simulink model "example_House_SFH15"  (R2013b)
settings: Solver=ode45  StartTime=-30*24*3600  StopTime=365*24*3600  RelTol=1e-3
libraries: carnot x5, simulink x3
settings Model: SimulationMode=accelerator  Creator=U_13.adm_zivi  LastModifiedBy=drhf
settings DataIOCC: SignalLoggingSaveFormat=ModelDataLogs
settings DebuggingCC: FcnCallInpInsideContextMsg=EnableAllAsWarning
settings GRTTargetCC: CombineOutputUpdateFcns=off  GRTInterface=on

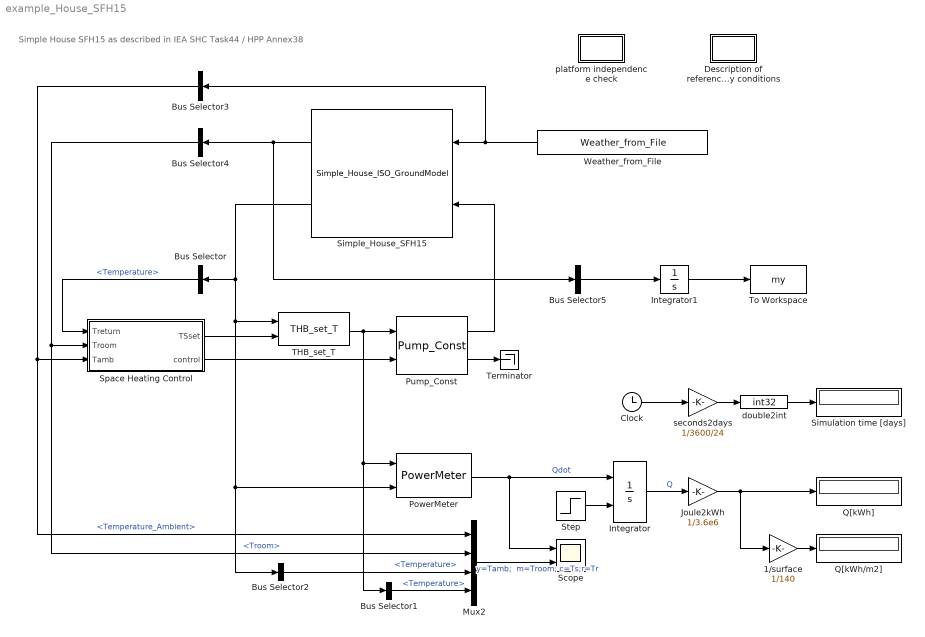
== system example_House_SFH15 ==
  note: Simple House SFH15 as described in IEA SHC Task44 / HPP Annex38
  1/surface : Gain  Gain=1/140
  Bus Selector : BusSelector  OutputSignals=Temperature
  Bus Selector1 : BusSelector  OutputSignals=Temperature
  Bus Selector2 : BusSelector  OutputSignals=Temperature
  Bus Selector3 : BusSelector  OutputSignals=Temperature_Ambient
  Bus Selector4 : BusSelector  OutputSignals=Troom
  Bus Selector5 : BusSelector  OutputSignals=Qdot  OutputAsBus=on
  Clock : Clock
  "Description of reference buidling and boundary conditions " : Subsystem
      settings: OpenFcn=|
      | filepath = fullfile(path_carnot('libsl'),'Load','Houses', 'Simple_House_ISO_GroundModel','specification');
      | 
      | open(fullfile(filepath, 'T44A38_Rep_C1_B_ReferenceBuildingDescription_Final_Revised_130906.pdf'));
      | open(fullfile(filepath, 'T44A38_Rep_C1_A_BoundaryConditions_Final_Revised_131108.pdf'));
      mask Display: disp('.pdf')
  Integrator : Integrator  ExternalReset=rising
  Integrator1 : Integrator
  Joule2kWh : Gain  Gain=1/3.6e6
  Mux2 : Mux
  PowerMeter : carnot/Control/PowerMeter
  Pump_Const : carnot/Hydraulics/Pump_Const  mdotmax=308/3600  dia=0.02  power=81  p0=3e5  fluid_id=Water  mix=0  UA=3  mcp=4000  tamb=20
  Q[kWh/m2] : Display
  Q[kWh] : Display
  Scope : Scope  NumInputPorts=2
      settings: TickLabels=on  YMin=-7.5~0  YMax=35~0.0019  Decimation=1000  SampleInput=on  SampleTime=3600*3
  Simple_House_SFH15 : carnot/Load/Houses/Simple_House_ISO_GroundModel  Ahabit=140  Hroom=2.6  Floorsize=[7 10]  UAwall=0.162*(54.6+26.4)+0.182*((45.7+56.0)*2 -(12+4+3+4))  UAneighbour=0  Uground=0.1  mc=0.5e6*140 % 0.5 MJ/m2/K  shade=0.75  tini=20  Awin=[12 4 3 4]  AziWin=[0 90 -180 -90]  Uwin="[1    1   1    1]*1.0"  Gwin="[1    1   1    1]*0.585*(1-0.15)"  vent=0.4  rec=0.6  heatload=1792  delta_t_nom=15  n_rad=1.1  mass_times_cap=40e6  dpcoeff=[10 100]
  Simulation time [days] : Display
  Space Heating Control : Subsystem  mask{Tset=20, Q_LOC=1792, Td_in=35, Td_out=30, Tambd=-10, n_rad=1.1}
      mask prompts: Tset "desired room Temperature [°C]"; Q_LOC "design heat load [W]"; Td_in "design inlet temperature of the heating system [°C]"; Td_out "design outlet temperature of the heating system [°C]"; Tambd "design outdoor temperature"; n_rad "radiatior exponent"
      mask init:
      | dTd = 0.5*(Td_in + Td_out) - Tset;
  Step : Step  Time=0  SampleTime=0
  THB_set_T : carnot/Source/Simple/THB_set_T
  Terminator : Terminator
  To Workspace : ToWorkspace  VariableName=my  SampleTime=3600
  Weather_from_File : carnot/Weather/Weather_from_File  file=DE_TRY2010_12_averageYear  ext=.mat
  double2int : DataTypeConversion  OutDataTypeStr=int32
  "platform independence check " : Subsystem
      settings: OpenFcn=open(fullfile(path_carnot('help'), 'pdf', 'Peter_Wintler_Dott_IEA_Task_44_Building_2014.pdf'));
      mask Display: disp('.pdf')
  seconds2days : Gain  Gain=1/3600/24
  wires:
  Space Heating Control/1(TSset) -> THB_set_T/2
  Space Heating Control/2(control) -> Pump_Const/2
  Weather_from_File/1 -> Bus Selector3/1, Simple_House_SFH15/1
  Pump_Const/1 -> Simple_House_SFH15/2
  Simple_House_SFH15/2 -> Bus Selector/1, Bus Selector2/1, PowerMeter/2, THB_set_T/1
  Bus Selector/1 -> Space Heating Control/1(Treturn)  "<Temperature>"
  Simple_House_SFH15/1 -> Bus Selector4/1, Bus Selector5/1
  Pump_Const/2 -> Terminator/1
  Bus Selector3/1 -> Space Heating Control/3(Tamb), Mux2/1  "<Temperature_Ambient>"
  Clock/1 -> seconds2days/1
  seconds2days/1 -> double2int/1
  double2int/1 -> Simulation time [days]/1
  Bus Selector2/1 -> Mux2/3  "<Temperature>"
  Bus Selector1/1 -> Mux2/4  "<Temperature>"
  PowerMeter/1 -> Integrator/1, Scope/1  "Qdot"
  1/surface/1 -> Q[kWh/m2]/1
  Integrator/1 -> Joule2kWh/1  "Q"
  THB_set_T/1 -> Bus Selector1/1, PowerMeter/1, Pump_Const/1
  Step/1 -> Integrator/2
  Mux2/1 -> Scope/2  "y=Tamb;  m=Troom; c=Ts;r=Tr"
  Joule2kWh/1 -> 1/surface/1, Q[kWh]/1
  Integrator1/1 -> To Workspace/1
  Bus Selector4/1 -> Mux2/2, Space Heating Control/2(Troom)  "<Troom>"
  Bus Selector5/1 -> Integrator1/1

== system example_House_SFH15/Description of reference buidling and boundary conditions  ==

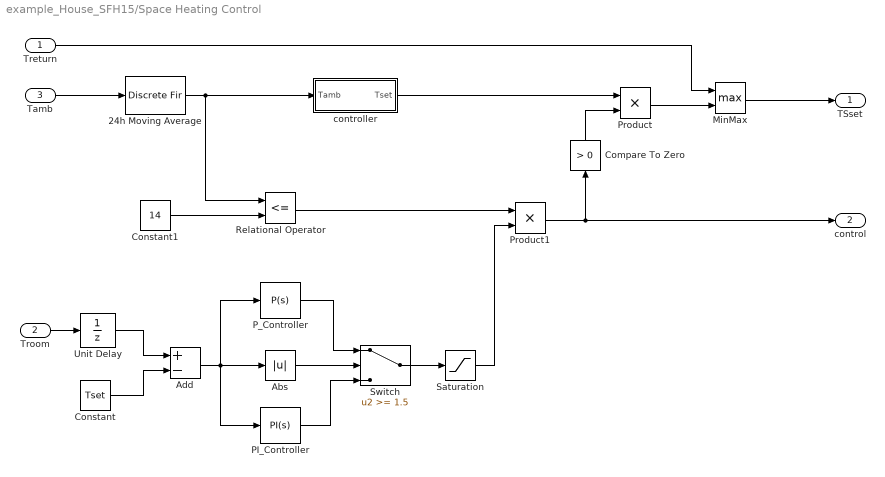
== system example_House_SFH15/Space Heating Control ==
  Treturn : Inport
  Troom : Inport  Port=2
  Tamb : Inport  Port=3
  24h Moving Average : DiscreteFir  Coefficients=ones(1,24)*(1/24)  SampleTime=3600  AccumDataTypeStr=Inherit: Same as product output  RndMeth=Nearest
  Abs : Abs
  Add : Sum  Inputs=+-
  Compare To Zero : simulink/Logic and Bit Operations/Compare To Zero  relop=>  OutDataTypeStr=boolean
  Constant : Constant  Value=Tset
  Constant1 : Constant  Value=14
  MinMax : MinMax  Function=max  Inputs=2
  PI_Controller : simulink/Continuous/PID Controller  Controller=PI  TimeDomain=Continuous-time  SampleTime=1  IntegratorMethod=Forward Euler  FilterMethod=Forward Euler  Form=Parallel  P=-0.8  I=-0.05/3600  D=0  N=100  InitialConditionSource=internal  InitialConditionForIntegrator=0  InitialConditionForFilter=0  ExternalReset=none  ZeroCross=off  LimitOutput=on  UpperSaturationLimit=1  LowerSaturationLimit=0  LinearizeAsGain=off  AntiWindupMode=back-calculation  Kb=1  TrackingMode=off  Kt=1  PParamMin=[]  PParamMax=[]  IParamMin=[]  IParamMax=[]  DParamMin=[]  DParamMax=[]  NParamMin=[]  NParamMax=[]  KbParamMin=[]  KbParamMax=[]  KtParamMin=[]  KtParamMax=[]  POutMin=[]  POutMax=[]  IOutMin=[]  IOutMax=[]  DOutMin=[]  DOutMax=[]  NOutMin=[]  NOutMax=[]  KbOutMin=[]  KbOutMax=[]  KtOutMin=[]  KtOutMax=[]  IntegratorOutMin=[]  IntegratorOutMax=[]  FilterOutMin=[]  FilterOutMax=[]  SumOutMin=[]  SumOutMax=[]  SumI1OutMin=[]  SumI1OutMax=[]  SumI2OutMin=[]  SumI2OutMax=[]  SumI3OutMin=[]  SumI3OutMax=[]  SumDOutMin=[]  SumDOutMax=[]  SaturationOutMin=[]  SaturationOutMax=[]  IntegratorContinuousStateAttributes=''  IntegratorStateMustResolveToSignalObject=off  IntegratorRTWStateStorageClass=Auto  FilterContinuousStateAttributes=''  FilterStateMustResolveToSignalObject=off  FilterRTWStateStorageClass=Auto
  P_Controller : simulink/Continuous/PID Controller  Controller=P  TimeDomain=Continuous-time  SampleTime=1  IntegratorMethod=Forward Euler  FilterMethod=Forward Euler  Form=Parallel  P=-0.5  I=1  D=0  N=100  InitialConditionSource=internal  InitialConditionForIntegrator=0  InitialConditionForFilter=0  ExternalReset=none  ZeroCross=off  LimitOutput=on  UpperSaturationLimit=1  LowerSaturationLimit=0  LinearizeAsGain=off  AntiWindupMode=none  Kb=1  TrackingMode=off  Kt=1  PParamMin=[]  PParamMax=[]  IParamMin=[]  IParamMax=[]  DParamMin=[]  DParamMax=[]  NParamMin=[]  NParamMax=[]  KbParamMin=[]  KbParamMax=[]  KtParamMin=[]  KtParamMax=[]  POutMin=[]  POutMax=[]  IOutMin=[]  IOutMax=[]  DOutMin=[]  DOutMax=[]  NOutMin=[]  NOutMax=[]  KbOutMin=[]  KbOutMax=[]  KtOutMin=[]  KtOutMax=[]  IntegratorOutMin=[]  IntegratorOutMax=[]  FilterOutMin=[]  FilterOutMax=[]  SumOutMin=[]  SumOutMax=[]  SumI1OutMin=[]  SumI1OutMax=[]  SumI2OutMin=[]  SumI2OutMax=[]  SumI3OutMin=[]  SumI3OutMax=[]  SumDOutMin=[]  SumDOutMax=[]  SaturationOutMin=[]  SaturationOutMax=[]  IntegratorContinuousStateAttributes=''  IntegratorStateMustResolveToSignalObject=off  IntegratorRTWStateStorageClass=Auto  FilterContinuousStateAttributes=''  FilterStateMustResolveToSignalObject=off  FilterRTWStateStorageClass=Auto
  Product : Product
  Product1 : Product
  Relational Operator : RelationalOperator  Operator=<=  OutDataTypeStr=boolean
  Saturation : Saturate  UpperLimit=1  LowerLimit=0  ZeroCross=off
  Switch : Switch  Threshold=1.5
  Unit Delay : UnitDelay  SampleTime=60
  controller : Subsystem
  TSset : Outport
  control : Outport  Port=2
  wires:
  Tamb/1 -> 24h Moving Average/1
  MinMax/1 -> TSset/1
  Troom/1 -> Unit Delay/1
  Constant1/1 -> Relational Operator/2
  Unit Delay/1 -> Add/1
  Constant/1 -> Add/2
  Add/1 -> P_Controller/1, PI_Controller/1, Abs/1
  Abs/1 -> Switch/2
  P_Controller/1 -> Switch/1
  PI_Controller/1 -> Switch/3
  Switch/1 -> Saturation/1
  Saturation/1 -> Product1/2
  Relational Operator/1 -> Product1/1
  Product/1 -> MinMax/2
  Treturn/1 -> MinMax/1
  Product1/1 -> control/1, Compare To Zero/1
  Compare To Zero/1 -> Product/2
  24h Moving Average/1 -> Relational Operator/1, controller/1(Tamb)
  controller/1(Tset) -> Product/1

== system example_House_SFH15/platform independence check  ==

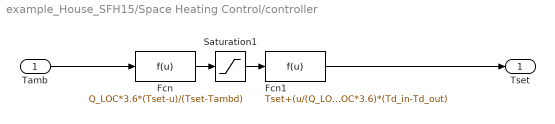
== system example_House_SFH15/Space Heating Control/controller ==
  Tamb : Inport
  Fcn : Fcn  Expr=Q_LOC*3.6*(Tset-u)/(Tset-Tambd)
  Fcn1 : Fcn  Expr=Tset+(u/(Q_LOC*3.6))^(1/n_rad)*dTd+u/(2*Q_LOC*3.6)*(Td_in-Td_out)
  Saturation1 : Saturate  UpperLimit=inf  LowerLimit=0
  Tset : Outport
  wires:
  Tamb/1 -> Fcn/1
  Fcn/1 -> Saturation1/1
  Fcn1/1 -> Tset/1
  Saturation1/1 -> Fcn1/1
